simulink model "yoshi_rover_linefollowing"  (R2013b)
settings: Solver=ode3  SolverMode=SingleTasking  StartTime=0.0  StopTime=inf  RelTol=1e-3
model workspace (MAT data in the model file):
  blc = -50
  brc = -50
  flc = 50
  frc = 50
  rc = 0
undefined symbols (not defined in the file): DiscIntNeverNeededParam, sigbuilder_block, SlDemoSign
libraries: arduinolib x13, simulink x9, battlebots_library x1
settings Model: SimulationMode=external  ExtModeTrigDuration=2  Creator=sbiagion  LastModifiedBy=abhayg
settings OptimizationCC: OptimizeModelRefInitCode=on  LifeSpan=1
settings DebuggingCC: SolverPrmCheckMsg=none
settings HardwareCC: ProdBitPerInt=16  ProdBitPerPointer=8  ProdIntDivRoundTo=Zero  ProdEndianess=LittleEndian  ProdWordSize=8  ProdHWDeviceType=Atmel->AVR
settings RTWCC: SystemTargetFile=realtime.tlc  GenerateMakefile=off  TemplateMakefile=realtime.tmf  Description=Run on Target Hardware  RTWVerbose=off  ProcessScript=realtime_make_rtw_hook
settings STFCustomTargetCC: TargetLibSuffix=.a  GenerateSampleERTMain=on  ERTCustomFileBanners=on  SupportNonInlinedSFcns=off  SupportVariableSizeSignals=on  MATLABClassNameForMDSCustomization=Simulink.SoftwareTarget.ERTCustomization  GRTInterface=off  SystemTargetFile=realtime.tlc
settings ERTTargetCC: CodeReplacementLibrary=ANSI_C  GenerateSampleERTMain=on  ParMdlRefBuildCompliant=off  CompOptLevelCompliant=off  ConcurrentExecutionCompliant=off  CombineOutputUpdateFcns=off  ERTFirstTimeCompliant=off  SupportContinuousTime=on  SupportVariableSizeSignals=on  ModelStepFunctionPrototypeControlCompliant=off  CPPClassGenCompliant=off  ExtMode=on  ExtModeTransport=3  ExtModeMexFile=ext_serial_win32_comm  ExtModeMexArgs=0 7 115200  InlinedParameterPlacement=NonHierarchical  ERTSrcFileBannerTemplate=realtime_code_template.cgt  ERTHdrFileBannerTemplate=realtime_code_template.cgt  ERTDataSrcFileTemplate=realtime_code_template.cgt  ERTDataHdrFileTemplate=realtime_code_template.cgt  ERTCustomFileTemplate=realtime_file_process.tlc

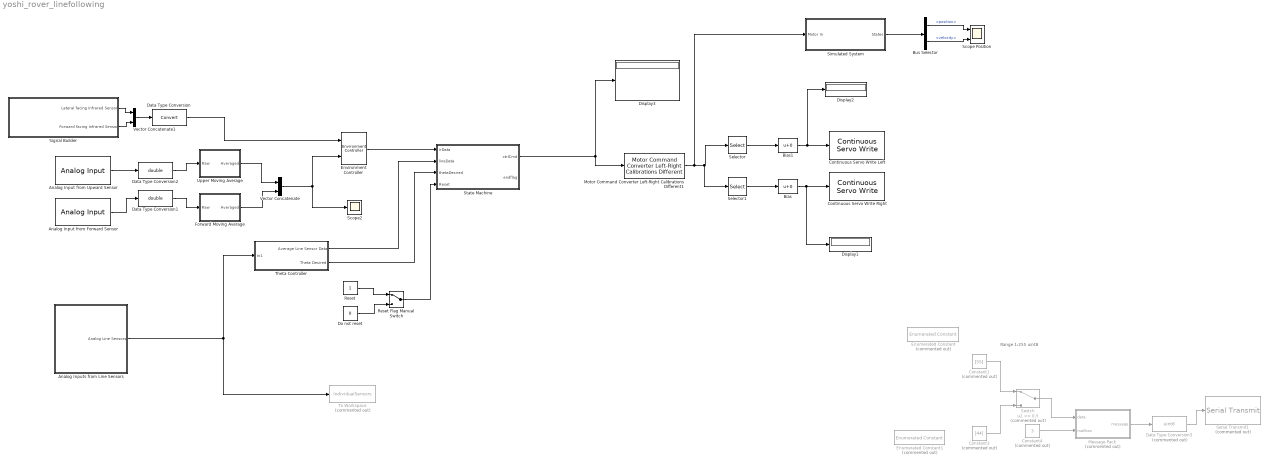
== system yoshi_rover_linefollowing ==
  note: Range 1:255 uint8
  Analog Input from Forward Sensor : arduinolib/Analog Input  pinNumber=1  sampleTime=0.01
  Analog Input from Upward Sensor : arduinolib/Analog Input  pinNumber=0  sampleTime=0.01
  Analog Inputs from Line Sensors : Subsystem
  Bias : Bias
  Bias1 : Bias
  Bus Selector : BusSelector  OutputSignals=position,velocity
  Constant1 : Constant  Commented=on  Value=[55]
  Constant3 : Constant  Commented=on  Value=[44]
  Constant4 : Constant  Commented=on  Value=3
  Continuous Servo Write Left : arduinolib/Continuous Servo Write  pinNumber=48
  Continuous Servo Write Right : arduinolib/Continuous Servo Write  pinNumber=49
  Data Type Conversion : DataTypeConversion
  Data Type Conversion1 : DataTypeConversion  OutDataTypeStr=double
  Data Type Conversion2 : DataTypeConversion  OutDataTypeStr=double
  Data Type Conversion3 : DataTypeConversion  Commented=on  OutDataTypeStr=uint8
  Display1 : Display
  Display2 : Display
  Display3 : Display
  Do not reset : Constant  Value=0
  Enumerated Constant : simulink/Sources/Enumerated Constant  Commented=on  OutDataTypeStr=Enum: SlDemoSign  Value=SlDemoSign.Positive  SampleTime=inf
  Enumerated Constant1 : simulink/Sources/Enumerated Constant  Commented=on  OutDataTypeStr=Enum: SlDemoSign  Value=SlDemoSign.Positive  SampleTime=inf
  Environment Controller : simulink/Signal Routing/Environment Controller
  Forward Moving Average : Subsystem
  Message Pack : Subsystem  Commented=on
  Motor Command Converter Left-Right Calibrations Different1 : battlebots_library/Motor Control/Motor Command Converter  Left-Right Calibrations Different  fcl=50  fcr=50  rc=0  bcl=-50  bcr=-50
  Reset : Constant
  Reset Flag Manual Switch : ManualSwitch
  Scope Position : Scope  NumInputPorts=2
      settings: ShowLegends=on  YMin=-5~-0.5  YMax=5~1  SaveName=ScopeData3
  Scope2 : Scope
      settings: ShowLegends=on  YMin=25  YMax=475  SaveName=ScopeData2
  Selector : Selector  InputPortWidth=2  IndexOptions=Index vector (dialog)  Indices=1  OutputSizes=1
  Selector1 : Selector  InputPortWidth=2  IndexOptions=Index vector (dialog)  Indices=2  OutputSizes=1
  Serial Transmit1 : arduinolib/Serial Transmit  Commented=on  portNumber=1
  Signal Builder : Subsystem  Tag=STV Subsys  LoadFcn=sigbuilder_block('load');  StartFcn=sigbuilder_block('start');  StopFcn=sigbuilder_block('stop');  ClipboardFcn=sigbuilder_block('clipboard');  mask(Sigbuilder block){}
      mask help: Simulink:masks:SigbuilderBlock_MD
      mask init:
      | if ~strcmp(get_param(bdroot(gcbh),'SimulationStatus'),'stopped') tuvar = sigbuilder_block('maskInit'); end
      settings: CopyFcn=sigbuilder_block('copy');  DeleteFcn=sigbuilder_block('delete');  ModelCloseFcn=sigbuilder_block('modelClose');  PreSaveFcn=sigbuilder_block('preSave');  PauseFcn=sigbuilder_block('pause');  ContinueFcn=sigbuilder_block('continue');  NameChangeFcn=sigbuilder_block('namechange');  OpenFcn=sigbuilder_block('open',[36 193.034 550.552 399.724 ]);  CloseFcn=sigbuilder_block('close');
      mask Display: plot(0, 0, 100, 100,[2, 2, 32, 32, 2], [68, 8, 8, 68, 68],[32, 2], [38, 38], [32, 19, 2],[53, 60, 44], [32, 17, 17, 2],[16, 16, 31, 31]);txt = getActiveGroup(gcbh);text(2, 100, txt,'verticalAlignment', 'top');
  Simulated System : Subsystem  AncestorBlock=battlebots_library/Simulation/Simulated System1  mask{max2vel=1, xm_initial_ft=0, ym_initial_ft=0, om_initial_rad=0, wheelbase_ft=1}
      mask prompts: max2vel "Gain to convert maximum command to velocity"; xm_initial_ft "Initial x position in ft"; ym_initial_ft "Initial y position in ft"; om_initial_rad "Initial orientation in radians"; wheelbase_ft "Wheelbase in ft"
      mask DialogControl DescTextVar Prompt: Rover Simulator
  State Machine : Stateflow chart  TreatAsAtomicUnit=on
  Switch : Switch  Commented=on  Threshold=0.5
  Theta Controller : Subsystem
  To Workspace : ToWorkspace  Commented=on  VariableName=IndividualSensors  SampleTime=-1  SaveFormat=Structure With Time
  Upper Moving Average : Subsystem
  Vector Concatenate : Concatenate
  Vector Concatenate1 : Concatenate
  wires:
  Analog Input from Upward Sensor/1 -> Data Type Conversion2/1
  Data Type Conversion/1 -> Environment Controller/1
  Signal Builder/2(Forward facing Infrared Sensor) -> Vector Concatenate1/2
  Signal Builder/1(Lateral facing Infrared Sensor) -> Vector Concatenate1/1
  Vector Concatenate1/1 -> Data Type Conversion/1
  Selector/1 -> Bias1/1
  Selector1/1 -> Bias/1
  Motor Command Converter Left-Right Calibrations Different1/1 -> Simulated System/1(Motor In), Selector1/1, Selector/1
  Vector Concatenate/1 -> Scope2/1, Environment Controller/2
  Analog Input from Forward Sensor/1 -> Data Type Conversion1/1
  Bias/1 -> Display1/1, Continuous Servo Write Right/1
  Bias1/1 -> Display2/1, Continuous Servo Write Left/1
  Simulated System/1(States) -> Bus Selector/1
  Bus Selector/1 -> Scope Position/1  "<position>"
  Bus Selector/2 -> Scope Position/2  "<velocity>"
  Data Type Conversion2/1 -> Upper Moving Average/1(Raw)
  Data Type Conversion1/1 -> Forward Moving Average/1(Raw)
  Forward Moving Average/1("Averaged ") -> Vector Concatenate/2
  Upper Moving Average/1(Averaged) -> Vector Concatenate/1
  Environment Controller/1 -> State Machine/1(irData)
  Reset Flag Manual Switch/1 -> State Machine/4(Reset)
  Reset/1 -> Reset Flag Manual Switch/1
  Do not reset/1 -> Reset Flag Manual Switch/2
  State Machine/1(ctrlCmd) -> Motor Command Converter Left-Right Calibrations Different1/1, Display3/1
  Analog Inputs from Line Sensors/1(Analog Line Sensors) -> To Workspace/1, Theta Controller/1(In1)
  Constant4/1 -> Message Pack/2(mailbox)
  Message Pack/1(message) -> Data Type Conversion3/1
  Constant1/1 -> Switch/1
  Constant3/1 -> Switch/3
  ? -> Switch/2
  Data Type Conversion3/1 -> Serial Transmit1/1
  Switch/1 -> Message Pack/1(data)
  Theta Controller/1(Average Line Sensor Data) -> State Machine/2(lineData)
  Theta Controller/2(Theta Desired) -> State Machine/3(thetaDesired)

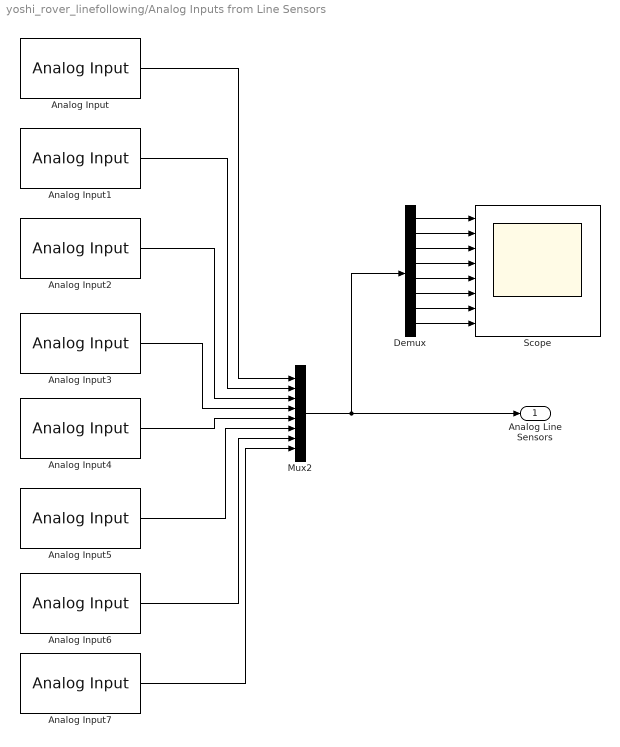
== system yoshi_rover_linefollowing/Analog Inputs from Line Sensors ==
  Analog Input : arduinolib/Analog Input  pinNumber=8  sampleTime=0.01
  Analog Input1 : arduinolib/Analog Input  pinNumber=9  sampleTime=0.01
  Analog Input2 : arduinolib/Analog Input  pinNumber=10  sampleTime=0.01
  Analog Input3 : arduinolib/Analog Input  pinNumber=11  sampleTime=0.01
  Analog Input4 : arduinolib/Analog Input  pinNumber=12  sampleTime=0.01
  Analog Input5 : arduinolib/Analog Input  pinNumber=13  sampleTime=0.01
  Analog Input6 : arduinolib/Analog Input  pinNumber=14  sampleTime=0.01
  Analog Input7 : arduinolib/Analog Input  pinNumber=15  sampleTime=0.01
  Demux : Demux  Outputs=8
  Mux2 : Mux  Inputs=8
  Scope : Scope  NumInputPorts=8
      settings: YMin=0~0~0~0~0~0~0~0  YMax=1300~1300~1300~1300~1300~1300~1300~1300
  Analog Line Sensors : Outport
  wires:
  Analog Input/1 -> Mux2/1
  Analog Input1/1 -> Mux2/2
  Analog Input2/1 -> Mux2/3
  Analog Input3/1 -> Mux2/4
  Analog Input5/1 -> Mux2/6
  Analog Input6/1 -> Mux2/7
  Analog Input7/1 -> Mux2/8
  Analog Input4/1 -> Mux2/5
  Mux2/1 -> Demux/1, Analog Line Sensors/1
  Demux/5 -> Scope/5
  Demux/4 -> Scope/4
  Demux/6 -> Scope/6
  Demux/3 -> Scope/3
  Demux/7 -> Scope/7
  Demux/8 -> Scope/8
  Demux/2 -> Scope/2
  Demux/1 -> Scope/1

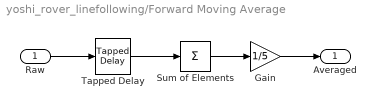
== system yoshi_rover_linefollowing/Forward Moving Average ==
  Raw : Inport
  Gain : Gain  Gain=1/5
  Sum of Elements : Sum  Inputs=+
  Tapped Delay : simulink/Discrete/Tapped Delay  vinit=0.0  samptime=-1  NumDelays=5  DelayOrder=Oldest  includeCurrent=off
  "Averaged " : Outport
  wires:
  Sum of Elements/1 -> Gain/1
  Tapped Delay/1 -> Sum of Elements/1
  Gain/1 -> "Averaged "/1
  Raw/1 -> Tapped Delay/1

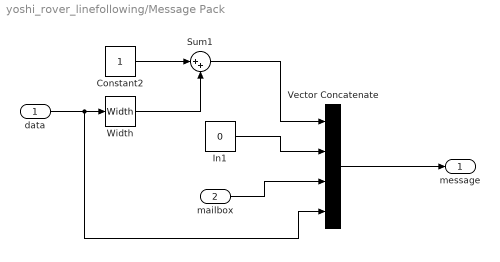
== system yoshi_rover_linefollowing/Message Pack ==
  data : Inport
  mailbox : Inport  Port=2
  Constant2 : Constant
  In1 : Constant  Value=0
  Sum1 : Sum  Inputs=|++
  Vector Concatenate : Concatenate  NumInputs=4
  Width : Width
  message : Outport
  wires:
  Constant2/1 -> Sum1/1
  In1/1 -> Vector Concatenate/2
  data/1 -> Vector Concatenate/4, Width/1
  Vector Concatenate/1 -> message/1
  mailbox/1 -> Vector Concatenate/3
  Sum1/1 -> Vector Concatenate/1
  Width/1 -> Sum1/2

== system yoshi_rover_linefollowing/Signal Builder ==
  Demux : Demux  Tag=STV Demux  Outputs=2
  FromWs : FromWorkspace  Tag=STV FromWs  VariableName=tuvar  OutputAfterFinalValue=Holding final value
      SigBuilderData=|
      | common.afterFinalStr = 'Hold final value'
      | common.sampleTime = '-1'
      | dataSet.timeRange = [0 20]
      | dataSet.name = 'Group 1'
      | sbobj.Groups.Name = 'Group 1'
      | sbobj.Groups.Signals(1).Name = 'Lateral facing Infrared Sensor'
      | sbobj.Groups.Signals(1).XData = [0 5 5 7 7 20]
      | sbobj.Groups.Signals(1).YData = [200 199.5 402 400 200 200]
      | sbobj.Groups.Signals(2).Name = 'Forward facing Infrared Sensor'
      | sbobj.Groups.Signals(2).XData = [0 12 16 20]
      | sbobj.Groups.Signals(2).YData = [200 200 450 496]
      | sbobj.Groups.TimeRange = [0 20]
  Lateral facing Infrared Sensor : Outport  Tag=STV Outport
  Forward facing Infrared Sensor : Outport  Tag=STV Outport  Port=2
  wires:
  Demux/1 -> Lateral facing Infrared Sensor/1
  FromWs/1 -> Demux/1
  Demux/2 -> Forward facing Infrared Sensor/1

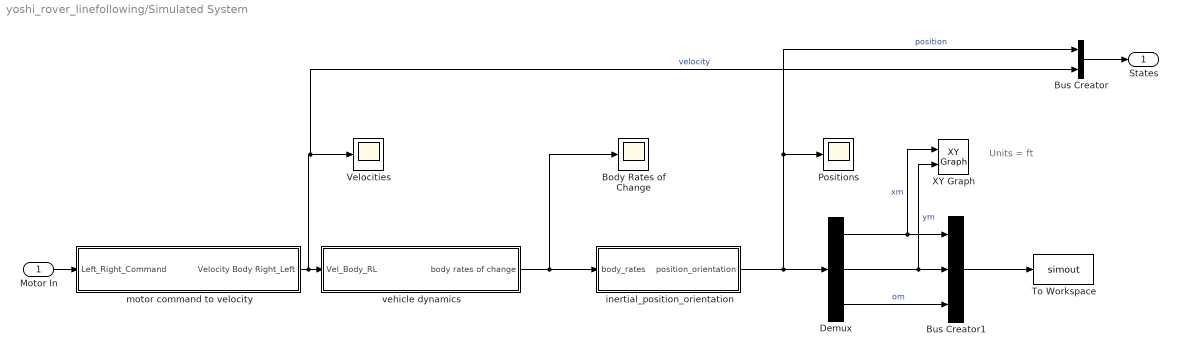
== system yoshi_rover_linefollowing/Simulated System ==
  note: Units = ft
  Motor In : Inport
  Body Rates of Change : Scope
      settings: ShowLegends=on  SaveName=ScopeData5
  Bus Creator : BusCreator  Inputs=2
  Bus Creator1 : BusCreator  Inputs=3
  Demux : Demux  Outputs=3
  Positions : Scope
      settings: ShowLegends=on  SaveName=ScopeData3
  To Workspace : ToWorkspace  VariableName=simout  SampleTime=-1  SaveFormat=Timeseries
  Velocities : Scope
      settings: ShowLegends=on  YMin=-1  YMax=1  SaveName=ScopeData4
  XY Graph : simulink/Sinks/XY Graph  xmin=-2  xmax=5  ymin=-5  ymax=5  st=1
  inertial_position_orientation : Subsystem
  motor command to velocity : Subsystem
  vehicle dynamics : Subsystem
  States : Outport
  wires:
  Bus Creator/1 -> States/1
  vehicle dynamics/1(body rates of change) -> Body Rates of Change/1, inertial_position_orientation/1(body_rates)
  inertial_position_orientation/1(position_orientation) -> Positions/1, Bus Creator/1, Demux/1  "position"
  motor command to velocity/1(Velocity Body Right_Left) -> Velocities/1, Bus Creator/2, vehicle dynamics/1(Vel_Body_RL)  "velocity"
  Motor In/1 -> motor command to velocity/1(Left_Right_Command)
  Demux/3 -> Bus Creator1/3  "om"
  Demux/2 -> Bus Creator1/2, XY Graph/2  "ym"
  Demux/1 -> Bus Creator1/1, XY Graph/1  "xm"
  Bus Creator1/1 -> To Workspace/1

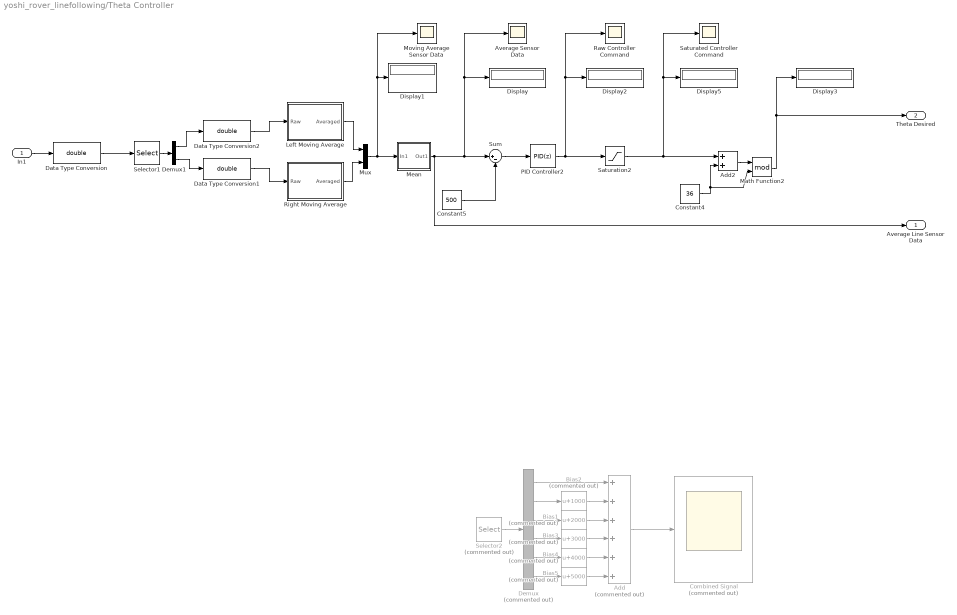
== system yoshi_rover_linefollowing/Theta Controller ==
  In1 : Inport
  Add : Sum  Commented=on  Inputs=++++++
  Add2 : Sum
  Average Sensor Data : Scope
      settings: YMin=0  YMax=2000  SaveName=ScopeData7
  Bias1 : Bias  Commented=on  Bias=2000
  Bias2 : Bias  Commented=on  Bias=1000
  Bias3 : Bias  Commented=on  Bias=3000
  Bias4 : Bias  Commented=on  Bias=4000
  Bias5 : Bias  Commented=on  Bias=5000
  Combined Signal : Scope  Commented=on
      settings: YMin=0  YMax=20000  SaveName=ScopeData6
  Constant4 : Constant  Value=36
  Constant5 : Constant  Value=500
  Data Type Conversion : DataTypeConversion  OutDataTypeStr=double
  Data Type Conversion1 : DataTypeConversion  OutDataTypeStr=double
  Data Type Conversion2 : DataTypeConversion  OutDataTypeStr=double
  Demux : Demux  Commented=on  Outputs=6
  Demux1 : Demux  Outputs=2
  Display{,1..3,5} (5 alike) : Display
  Left Moving Average : Subsystem
  Math Function2 : Math  Operator=mod  SaturateOnIntegerOverflow=on
  Mean : Subsystem
  Moving Average Sensor Data : Scope
      settings: YMin=0  YMax=2000
  Mux : Mux  Inputs=2
  PID Controller2 : simulink/Continuous/PID Controller  Controller=PID  TimeDomain=Discrete-time  SampleTime=-1  IntegratorMethod=Forward Euler  FilterMethod=Forward Euler  Form=Parallel  P=-1/30  I=0  D=-1/1000  N=100  InitialConditionSource=internal  InitialConditionForIntegrator=0  InitialConditionForFilter=0  ExternalReset=none  LimitOutput=off  UpperSaturationLimit=inf  LowerSaturationLimit=-inf  LinearizeAsGain=on  AntiWindupMode=none  Kb=1  TrackingMode=off  Kt=1  PParamMin=[]  PParamMax=[]  IParamMin=[]  IParamMax=[]  DParamMin=[]  DParamMax=[]  NParamMin=[]  NParamMax=[]  KbParamMin=[]  KbParamMax=[]  KtParamMin=[]  KtParamMax=[]  POutMin=[]  POutMax=[]  IOutMin=[]  IOutMax=[]  DOutMin=[]  DOutMax=[]  NOutMin=[]  NOutMax=[]  KbOutMin=[]  KbOutMax=[]  KtOutMin=[]  KtOutMax=[]  IntegratorOutMin=[]  IntegratorOutMax=[]  FilterOutMin=[]  FilterOutMax=[]  SumOutMin=[]  SumOutMax=[]  SumI1OutMin=[]  SumI1OutMax=[]  SumI2OutMin=[]  SumI2OutMax=[]  SumI3OutMin=[]  SumI3OutMax=[]  SumDOutMin=[]  SumDOutMax=[]  SaturationOutMin=[]  SaturationOutMax=[]  IntegratorContinuousStateAttributes=''  IntegratorStateMustResolveToSignalObject=off  IntegratorRTWStateStorageClass=Auto  FilterContinuousStateAttributes=''  FilterStateMustResolveToSignalObject=off  FilterRTWStateStorageClass=Auto
  Raw Controller Command : Scope
      settings: YMin=-20  YMax=20  SaveName=ScopeData8
  Right Moving Average : Subsystem
  Saturated Controller Command : Scope
      settings: YMin=-9  YMax=9  SaveName=ScopeData9
  Saturation2 : Saturate  UpperLimit=7  LowerLimit=-7
  Selector1 : Selector  InputPortWidth=8  IndexOptions=Index vector (dialog)  Indices=5:6  OutputSizes=1
  Selector2 : Selector  Commented=on  InputPortWidth=8  IndexOptions=Index vector (dialog)  Indices=2:7  OutputSizes=1
  Sum : Sum  Inputs=|+-
  Average Line Sensor Data : Outport
  Theta Desired : Outport  Port=2
  wires:
  Math Function2/1 -> Theta Desired/1, Display3/1
  ? -> Selector2/1
  Selector2/1 -> Demux/1
  Demux/2 -> Bias2/1
  Demux/3 -> Bias1/1
  Demux/4 -> Bias3/1
  Demux/5 -> Bias4/1
  Demux/6 -> Bias5/1
  Demux/1 -> Add/1
  Bias2/1 -> Add/2
  Bias1/1 -> Add/3
  Bias3/1 -> Add/4
  Bias4/1 -> Add/5
  Bias5/1 -> Add/6
  Add/1 -> Combined Signal/1
  In1/1 -> Data Type Conversion/1
  PID Controller2/1 -> Raw Controller Command/1, Display2/1, Saturation2/1
  Saturation2/1 -> Saturated Controller Command/1, Display5/1, Add2/1
  Constant4/1 -> Add2/2, Math Function2/2
  Add2/1 -> Math Function2/1
  Data Type Conversion/1 -> Selector1/1
  Constant5/1 -> Sum/2
  Sum/1 -> PID Controller2/1
  Demux1/1 -> Data Type Conversion2/1
  Demux1/2 -> Data Type Conversion1/1
  Data Type Conversion2/1 -> Left Moving Average/1(Raw)
  Data Type Conversion1/1 -> Right Moving Average/1(Raw)
  Right Moving Average/1("Averaged ") -> Mux/2
  Left Moving Average/1(Averaged) -> Mux/1
  Mux/1 -> Moving Average Sensor Data/1, Display1/1, Mean/1(In1)
  Selector1/1 -> Demux1/1
  Mean/1(Out1) -> Average Line Sensor Data/1, Average Sensor Data/1, Display/1, Sum/1

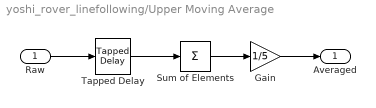
== system yoshi_rover_linefollowing/Upper Moving Average ==
  Raw : Inport
  Gain : Gain  Gain=1/5
  Sum of Elements : Sum  Inputs=+
  Tapped Delay : simulink/Discrete/Tapped Delay  vinit=0.0  samptime=-1  NumDelays=5  DelayOrder=Oldest  includeCurrent=off
  Averaged : Outport
  wires:
  Raw/1 -> Tapped Delay/1
  Gain/1 -> Averaged/1
  Tapped Delay/1 -> Sum of Elements/1
  Sum of Elements/1 -> Gain/1

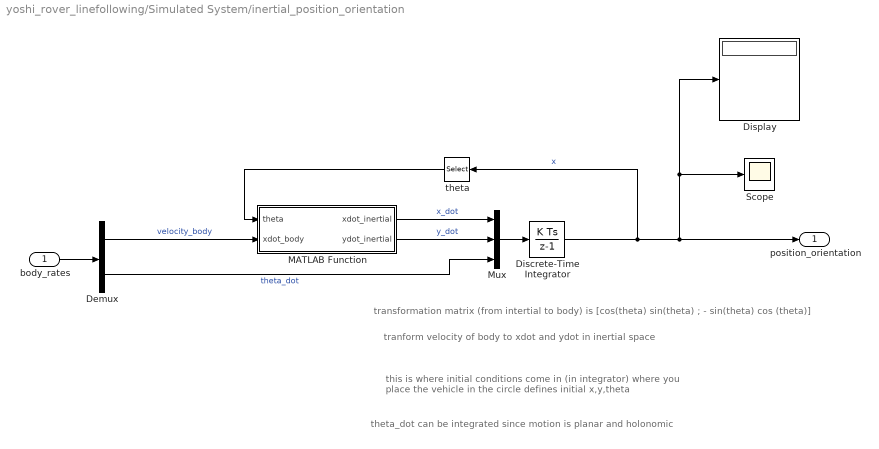
== system yoshi_rover_linefollowing/Simulated System/inertial_position_orientation ==
  note: transformation matrix (from intertial to body) is [cos(theta) sin(theta) ; - sin(theta) cos (theta)]
  note: tranform velocity of body to xdot and ydot in inertial space
  note: this is where initial conditions come in (in integrator)
      | where you place the vehicle in the circle defines initial x,y,theta
  note: theta_dot can be integrated since motion is planar and holonomic
  body_rates : Inport
  Demux : Demux  Outputs=2
  Discrete-Time Integrator : DiscreteIntegrator  InitialCondition=[xm_initial_ft ym_initial_ft om_initial_rad]  SampleTime=-1  ICPrevOutput=DiscIntNeverNeededParam  ICPrevScaledInput=DiscIntNeverNeededParam
  Display : Display
  MATLAB Function : MATLAB Function  TreatAsAtomicUnit=on
  Mux : Mux  Inputs=3
  Scope : Scope
      settings: ShowLegends=on  YMin=-2  YMax=32  SaveName=ScopeData2
  theta : Selector  InputPortWidth=3  IndexOptions=Index vector (dialog)  Indices=[3]  OutputSizes=1
  position_orientation : Outport
  wires:
  MATLAB Function/1(xdot_inertial) -> Mux/1  "x_dot"
  MATLAB Function/2(ydot_inertial) -> Mux/2  "y_dot"
  Demux/2 -> Mux/3  "theta_dot"
  Demux/1 -> MATLAB Function/2(xdot_body)  "velocity_body"
  theta/1 -> MATLAB Function/1(theta)
  Mux/1 -> Discrete-Time Integrator/1
  Discrete-Time Integrator/1 -> position_orientation/1, Display/1, Scope/1, theta/1  "x"
  body_rates/1 -> Demux/1

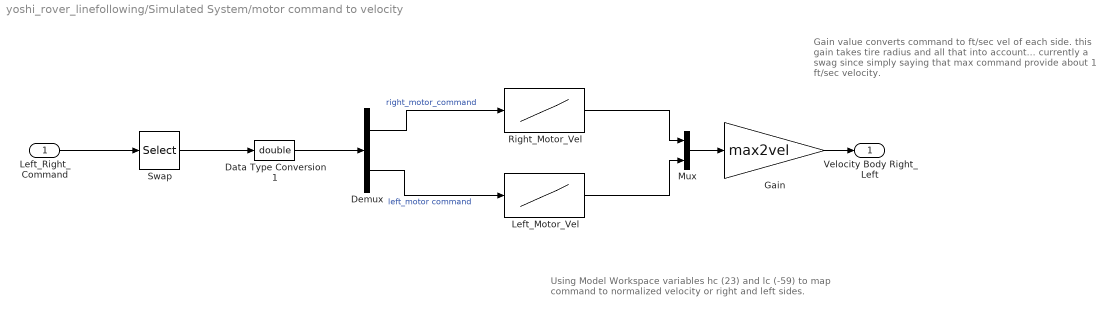
== system yoshi_rover_linefollowing/Simulated System/motor command to velocity ==
  note: Using Model Workspace variables hc (23) and lc (-59)
      | to map command to normalized velocity or right and left sides.
  note: Gain value converts command to ft/sec vel
      | of each side.  this gain takes tire radius and all that
      | into account... currently a swag since simply saying that max
      | command provide about 1 ft/sec velocity.
  Left_Right_Command : Inport
  Data Type Conversion1 : DataTypeConversion  OutDataTypeStr=double
  Demux : Demux  Outputs=2
  Gain : Gain  Gain=max2vel  ParamDataTypeStr=single  OutDataTypeStr=double
  Left_Motor_Vel : Lookup_n-D  NumberOfTableDimensions=1  BreakpointsForDimension1=[blc rc flc]  Table=[-1 0 1]  RndMeth=Simplest  InputSameDT=on
  Mux : Mux  Inputs=2
  Right_Motor_Vel : Lookup_n-D  NumberOfTableDimensions=1  BreakpointsForDimension1=[brc rc frc]  Table=[-1 0 1]  RndMeth=Simplest  InputSameDT=on
  Swap : Selector  InputPortWidth=2  IndexOptions=Index vector (dialog)  Indices=[2 1]  OutputSizes=1
  Velocity Body Right_Left : Outport  OutDataTypeStr=double
  wires:
  Data Type Conversion1/1 -> Demux/1
  Swap/1 -> Data Type Conversion1/1
  Demux/2 -> Left_Motor_Vel/1  "left_motor command"
  Demux/1 -> Right_Motor_Vel/1  "right_motor_command"
  Left_Right_Command/1 -> Swap/1
  Mux/1 -> Gain/1
  Right_Motor_Vel/1 -> Mux/1
  Left_Motor_Vel/1 -> Mux/2
  Gain/1 -> Velocity Body Right_Left/1

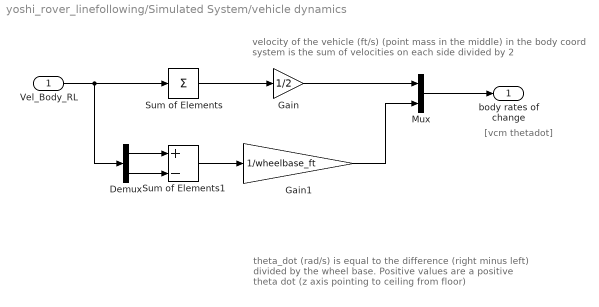
== system yoshi_rover_linefollowing/Simulated System/vehicle dynamics ==
  note: [vcm thetadot]
  note: velocity of the vehicle (ft/s) (point mass in the middle) in the body coord
      | system is the sum of velocities on each side divided by 2
  note: theta_dot (rad/s) is equal to the difference (right minus left)
      | divided by the wheel base.  Positive values are a
      | positive theta dot (z axis pointing to ceiling from floor)
  Vel_Body_RL : Inport
  Demux : Demux  Outputs=2
  Gain : Gain  Gain=1/2
  Gain1 : Gain  Gain=1/wheelbase_ft
  Mux : Mux  Inputs=2
  Sum of Elements : Sum  Inputs=+
  Sum of Elements1 : Sum  Inputs=+-
  body rates of change : Outport
  wires:
  Gain1/1 -> Mux/2
  Sum of Elements1/1 -> Gain1/1
  Demux/2 -> Sum of Elements1/2
  Demux/1 -> Sum of Elements1/1
  Gain/1 -> Mux/1
  Mux/1 -> body rates of change/1
  Sum of Elements/1 -> Gain/1
  Vel_Body_RL/1 -> Sum of Elements/1, Demux/1

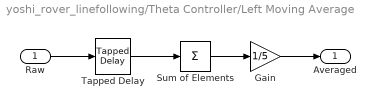
== system yoshi_rover_linefollowing/Theta Controller/Left Moving Average ==
  Raw : Inport
  Gain : Gain  Gain=1/5
  Sum of Elements : Sum  Inputs=+
  Tapped Delay : simulink/Discrete/Tapped Delay  vinit=0.0  samptime=-1  NumDelays=5  DelayOrder=Oldest  includeCurrent=off
  Averaged : Outport
  wires:
  Raw/1 -> Tapped Delay/1
  Gain/1 -> Averaged/1
  Tapped Delay/1 -> Sum of Elements/1
  Sum of Elements/1 -> Gain/1

== system yoshi_rover_linefollowing/Theta Controller/Mean ==
  In1 : Inport
  Gain : Gain  Gain=1/2
  Sum of Elements : Sum  Inputs=+
  Out1 : Outport
  wires:
  In1/1 -> Sum of Elements/1
  Sum of Elements/1 -> Gain/1
  Gain/1 -> Out1/1

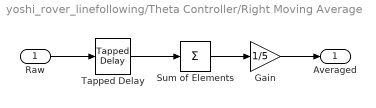
== system yoshi_rover_linefollowing/Theta Controller/Right Moving Average ==
  Raw : Inport
  Gain : Gain  Gain=1/5
  Sum of Elements : Sum  Inputs=+
  Tapped Delay : simulink/Discrete/Tapped Delay  vinit=0.0  samptime=-1  NumDelays=5  DelayOrder=Oldest  includeCurrent=off
  "Averaged " : Outport
  wires:
  Sum of Elements/1 -> Gain/1
  Tapped Delay/1 -> Sum of Elements/1
  Gain/1 -> "Averaged "/1
  Raw/1 -> Tapped Delay/1

== matlab function yoshi_rover_linefollowing/Simulated System/inertial_position_orientation/MATLAB Function ==
  data: theta input; xdot_inertial output; xdot_body input; ydot_inertial output
function [xdot_inertial, ydot_inertial]  = fcn(theta, xdot_body)
%#codegen

% transformation from intertial to body
T_bi = [cos(theta) sin(theta);
        -sin(theta) cos(theta)];
    
% note transpose of T since moving from body to inertial
vel_i = T_bi'*[xdot_body;0];

xdot_inertial = vel_i(1);
ydot_inertial = vel_i(2);

== stateflow chart yoshi_rover_linefollowing/State Machine ==
  state waitForMario
    en, du:
    ctrlCmd=[0 0];
    endflag = 0;
  note: 1.5 0
  state SlowDown
    en, du:
    ctrlCmd=[2.5 thetaDesired];
  state MoveForward
    entry:
    note: % if far from line for 0.5 seconds, enter state
    state FarFromLine
      state TurnLeft
        entry:
        ctrlCmd = [4 9];
      state MoveForwardSlowly
        entry:
        ctrlCmd = [2 0];
      (default) -> TurnLeft
      TurnLeft -> MoveForwardSlowly : [after(0.5,sec)]
      MoveForwardSlowly -> TurnLeft : [after(0.1,sec)]
    state CloseToLine
      en,du:
      ctrlCmd=[3 thetaDesired];
    state MaybeFarFromLine
      en,du:
      count = count+1;
    state TurnRight
      entry:
      ctrlCmd = [4 27];
    (default) -> CloseToLine
    MaybeFarFromLine -> FarFromLine [order 2] : [count>50]
    CloseToLine -> MaybeFarFromLine : [thetaDesired == 7]
    MaybeFarFromLine -> CloseToLine [order 1] : [thetaDesired ~=7]{count = 0;}
    TurnRight -> CloseToLine : after(0.5,sec)
    FarFromLine -> TurnRight : [thetaDesired ~=7]
  state Stop
    entry:
    ctrlCmd=[0 0];
    endflag = 1;
  state wait
  (default) -> waitForMario
  wait -> MoveForward : %[after(3,sec)]
  waitForMario -> wait : [irData(1)>300]
  SlowDown -> Stop : [irData(2)>440]
  MoveForward -> SlowDown : [irData(2)>300]
  Stop -> waitForMario : [Reset == 1]
  data: irData input; lineData input; thetaDesired input; ctrlCmd output double size=[1 2]; Reset input size=1; endflag output; count local
